simulink model "LPVT_CollectivePitch_50"  (R2018a)
settings: Solver=FixedStepAuto  StartTime=0.0  StopTime=FA.TMax  FixedStep=FA.DT  RelTol=1e-3  EnableMultiTasking=on
undefined symbols (not defined in the file or in its folder): Control, DiscIntNeverNeededParam, FA, OutList, Parameters, PitchControlParams, rpm2radps, S_ConstTq, S_LowBPLim, strmatch, TorqueControlParams
libraries: simulink_extras x1
settings Model: ExtModeTrigMode=oneshot  ExtModeArmWhenConnect=off  Creator=Dana Martin  LastModifiedBy=dmartin
settings DataIOCC: SaveFormat=Array  SaveOutput=off  InspectSignalLogs=on  SignalLoggingName=sigsOut  OutputTimes=[0:500]/50
settings OptimizationCC: BooleanDataType=off  ExpressionDepthLimit=2147483647  InitFltsAndDblsToZero=on  LifeSpan=inf
settings DebuggingCC: SignalRangeChecking=warning  AlgebraicLoopMsg=error  SaveWithParameterizedLinksMsg=none  UnderspecifiedInitializationDetection=Classic  MergeDetectMultiDrivingBlocksExec=none  SignalResolutionControl=TryResolveAllWithWarning  TimeAdjustmentMsg=warning  MultiTaskDSMMsg=warning  MultiTaskCondExecSysMsg=warning  ParameterUnderflowMsg=warning  UnderSpecifiedDataTypeMsg=warning  UnnecessaryDatatypeConvMsg=warning  VectorMatrixConversionMsg=warning  FcnCallInpInsideContextMsg=warning  SignalLabelMismatchMsg=warning  SFcnCompatibilityMsg=warning  UniqueDataStoreMsg=warning  AllowSymbolicDim=off  ModelReferenceIOMsg=warning  ModelReferenceVersionMismatchMessage=warning  ModelReferenceIOMismatchMessage=warning  StateNameClashWarn=warning  StrictBusMsg=WarnOnBusTreatedAsVector  NonBusSignalsTreatedAsBus=warning  SFUnexpectedBacktrackingDiag=warning  SFNoUnconditionalDefaultTransitionDiag=warning  SFExecutionAtInitializationDiag=none
settings HardwareCC: ProdBitPerPointer=32  ProdBitPerSizeT=32  ProdBitPerPtrDiffT=32  ProdLargestAtomicFloat=None  ProdIntDivRoundTo=Undefined  ProdEndianess=Unspecified  ProdWordSize=32  ProdHWDeviceType=32-bit Generic  TargetBitPerPointer=64  TargetBitPerSizeT=64  TargetBitPerPtrDiffT=64  TargetLongLongMode=on  TargetIntDivRoundTo=Zero  TargetEndianess=LittleEndian  TargetWordSize=64  TargetHWDeviceType=MATLAB Host  ProdEqTarget=off
settings ModelReferenceCC: PropagateSignalLabelsOutOfModel=off
settings CodeAppCC: StateflowObjectComments=on
settings GRTTargetCC: TargetFcnLib=ansi_tfl_tmw.mat  TargetLangStandard=C89/C90 (ANSI)  ModelReferenceCompliant=off  GeneratePreprocessorConditionals=Disable all  CombineOutputUpdateFcns=off  GRTInterface=on
settings ConfigComp: CovMetricSettings=dw  CovHtmlReporting=on  CovSaveCumulativeToWorkspaceVar=on  CovSaveSingleToWorkspaceVar=on  CovExternalEMLEnable=off  CovSFcnEnable=off

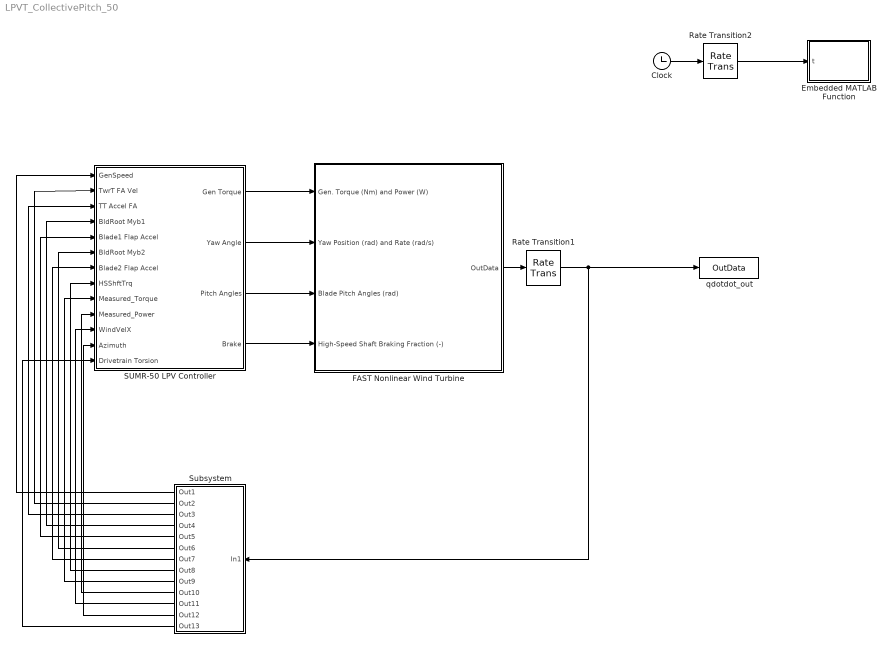
== system LPVT_CollectivePitch_50 ==
  Clock : Clock
  Embedded MATLAB Function : MATLAB Function  TreatAsAtomicUnit=on
  FAST Nonlinear Wind Turbine : Subsystem  mask(FAST Nonlinear Wind Turbine){}
      mask help: This block contains the FAST S-Function.
      mask init:
      | clear FAST_SFunc
  Rate Transition1 : RateTransition
  Rate Transition2 : RateTransition
  SUMR-50 LPV Controller : Subsystem
  Subsystem : Subsystem
  qdotdot_out : ToWorkspace  VariableName=OutData  SaveFormat=Structure With Time  SampleTime=-1
  wires:
  SUMR-50 LPV Controller/1(Gen Torque) -> FAST Nonlinear Wind Turbine/1(Gen. Torque (Nm) and Power (W))
  SUMR-50 LPV Controller/3(Pitch Angles) -> FAST Nonlinear Wind Turbine/3(Blade Pitch Angles (rad))
  SUMR-50 LPV Controller/2(Yaw Angle) -> FAST Nonlinear Wind Turbine/2(Yaw Position (rad) and Rate (rad/s))
  SUMR-50 LPV Controller/4(Brake) -> FAST Nonlinear Wind Turbine/4(High-Speed Shaft Braking Fraction (-))
  Rate Transition1/1 -> Subsystem/1(In1), qdotdot_out/1
  FAST Nonlinear Wind Turbine/1(OutData) -> Rate Transition1/1
  Subsystem/1(Out1) -> SUMR-50 LPV Controller/1(GenSpeed)
  Subsystem/2(Out2) -> SUMR-50 LPV Controller/2(TwrT FA Vel)
  Subsystem/3(Out3) -> SUMR-50 LPV Controller/3(TT Accel FA)
  Subsystem/4(Out4) -> SUMR-50 LPV Controller/4(BldRoot Myb1)
  Subsystem/5(Out5) -> SUMR-50 LPV Controller/5(Blade1 Flap Accel)
  Subsystem/6(Out6) -> SUMR-50 LPV Controller/6(BldRoot Myb2)
  Subsystem/7(Out7) -> SUMR-50 LPV Controller/7(Blade2 Flap Accel)
  Subsystem/8(Out8) -> SUMR-50 LPV Controller/8(HSShftTrq)
  Subsystem/9(Out9) -> SUMR-50 LPV Controller/9(Measured_Torque)
  Subsystem/10(Out10) -> SUMR-50 LPV Controller/10(Measured_Power)
  Subsystem/11(Out11) -> SUMR-50 LPV Controller/11(WindVelX)
  Subsystem/12(Out12) -> SUMR-50 LPV Controller/12(Azimuth)
  Clock/1 -> Rate Transition2/1
  Rate Transition2/1 -> Embedded MATLAB Function/1(t)
  Subsystem/13(Out13) -> SUMR-50 LPV Controller/13(Drivetrain Torsion)

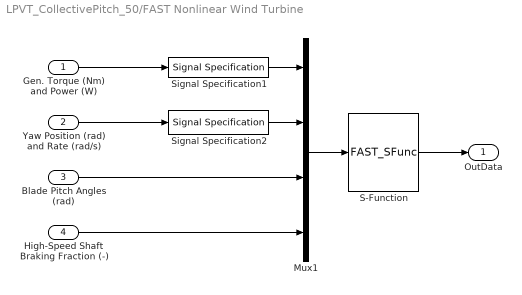
== system LPVT_CollectivePitch_50/FAST Nonlinear Wind Turbine ==
  Gen. Torque (Nm) and Power (W) : Inport
  Yaw Position (rad) and Rate (rad/s) : Inport  Port=2
  Blade Pitch Angles (rad) : Inport  Port=3
  High-Speed Shaft Braking Fraction (-) : Inport  Port=4
  Mux1 : Mux
  S-Function : S-Function  FunctionName=FAST_SFunc  Parameters=FAST_InputFileName, FA.TMax, 0  SFunctionDeploymentMode=off  EnableBusSupport=off
  Signal Specification1 : SignalSpecification  OutDataTypeStr=double  Dimensions=2
  Signal Specification2 : SignalSpecification  OutDataTypeStr=double  Dimensions=2
  OutData : Outport
  wires:
  Gen. Torque (Nm) and Power (W)/1 -> Signal Specification1/1
  S-Function/1 -> OutData/1
  Mux1/1 -> S-Function/1
  Blade Pitch Angles (rad)/1 -> Mux1/3
  Yaw Position (rad) and Rate (rad/s)/1 -> Signal Specification2/1
  Signal Specification1/1 -> Mux1/1
  Signal Specification2/1 -> Mux1/2
  High-Speed Shaft Braking Fraction (-)/1 -> Mux1/4

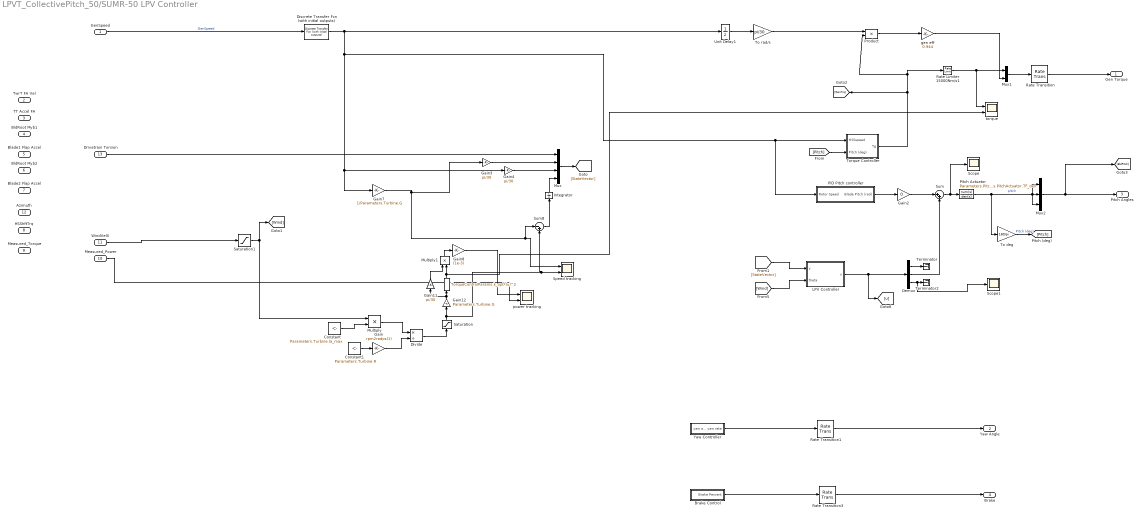
== system LPVT_CollectivePitch_50/SUMR-50 LPV Controller ==
  GenSpeed : Inport
  TwrT FA Vel : Inport  Port=2
  TT Accel FA : Inport  Port=3
  BldRoot Myb1 : Inport  Port=4
  Blade1 Flap Accel : Inport  Port=5
  BldRoot Myb2 : Inport  Port=6
  Blade2 Flap Accel : Inport  Port=7
  HSShftTrq : Inport  Port=8
  Measured_Torque : Inport  Port=9
  Measured_Power : Inport  Port=10
  WindVelX : Inport  Port=11
  Azimuth : Inport  Port=12
  Drivetrain Torsion : Inport  Port=13
  " " : Fcn  Expr=TorqueControlParams.k_opt*(u)^2
  Brake Control : Subsystem
  Constant : Constant  Value=Parameters.Turbine.la_max  SampleTime=FA.DT
  Constant1 : Constant  Value=Parameters.Turbine.R
  Demux : Demux  Outputs=3
  Discrete Transfer Fcn (with initial outputs) : simulink_extras/Additional Discrete/Discrete Transfer Fcn (with initial outputs)  N=Parameters.LPF.LPnum  D=Parameters.LPF.LPden  U0=Parameters.Turbine.IC.Wg  Y0=Parameters.Turbine.IC.Wg  TS=FA.DT
      settings: SourceProductName=Simulink  SourceProductBaseCode=SL
  Divide : Product  Inputs=*/
  Gain : Gain  Gain=rpm2radps(1)
  Gain11 : Gain  Gain=pi/30
  Gain12 : Gain  Gain=Parameters.Turbine.G
  Gain2 : Gain  Gain=0
  Gain3 : Gain  Gain=pi/30
  Gain4 : Gain  Gain=pi/30
  Gain7 : Gain  Gain=1/Parameters.Turbine.G
  Gain8 : Gain  Gain=(1e-3)
  Integrator : Integrator
  LPV Controller : Subsystem  TreatAsAtomicUnit=on
      settings: MinAlgLoopOccurrences=on
  Multiply : Product
  Multiply1 : Product
  Mux : Mux
  Mux1 : Mux  Inputs=2
  Mux2 : Mux  Inputs=3
  PID Pitch controller : Subsystem
      settings: MinAlgLoopOccurrences=on
  Pitch Actuator : TransferFcn  Numerator=Parameters.PitchActuator.TF_num  Denominator=Parameters.PitchActuator.TF_den
  Product : Product  RndMeth=Zero
  Rate Limiter 15000Nm/s1 : RateLimiter  RisingSlewLimit=15000  FallingSlewLimit=-15000  SampleTimeMode=inherited
  Rate Transition : RateTransition  InitialCondition=Parameters.Turbine.IC.Tg
  Rate Transition1 : RateTransition
  Rate Transition3 : RateTransition
  Saturation : Saturate  UpperLimit=Parameters.Turbine.wr_rated  LowerLimit=0
  Saturation1 : Saturate  UpperLimit=25  LowerLimit=0
  Scope : Scope
  Scope1 : Scope
  Speed tracking : Scope  NumInputPorts=2
  Sum : Sum  Inputs=|++
  Sum8 : Sum  Inputs=|-+
  Terminator : Terminator
  Terminator2 : Terminator
  To deg : Gain  Gain=180/pi
  To rad/s : Gain  Gain=pi/30
  Torque Controller : Subsystem
  Unit Delay1 : UnitDelay  InitialCondition=Parameters.Turbine.IC.Wg  SampleTime=FA.DT
  Yaw Controller : Subsystem
  gen eff : Gain  Gain=0.944
  power tracking : Scope  NumInputPorts=2
  torque : Scope  NumInputPorts=2
  Gen Torque : Outport
  Yaw Angle : Outport  Port=2
  Pitch Angles : Outport  Port=3
  Brake : Outport  Port=4
  wires:
  Mux1/1 -> Rate Transition/1
  Product/1 -> gen eff/1
  Unit Delay1/1 -> To rad/s/1
  To rad/s/1 -> Product/1
  gen eff/1 -> Mux1/2
  GenSpeed/1 -> Discrete Transfer Fcn (with initial outputs)/1  "GenSpeed"
  Yaw Controller/1(yaw and yaw rate) -> Rate Transition1/1
  Brake Control/1(Brake Percent) -> Rate Transition3/1
  Rate Transition3/1 -> Brake/1
  Rate Transition1/1 -> Yaw Angle/1
  Constant/1 -> Multiply/2
  Multiply/1 -> Divide/1
  Constant1/1 -> Gain/1
  Gain/1 -> Divide/2
  LPV Controller/1(u) -> Demux/1, [u]
  Mux2/1 -> [BldPitch], Pitch Angles/1
  Rate Transition/1 -> Gen Torque/1
  WindVelX/1 -> Saturation1/1
  Multiply1/1 -> Gain8/1
  Gain11/1 -> Multiply1/1
  Divide/1 -> Saturation/1
  Gain12/1 -> Gain11/1, " "/1
  Saturation1/1 -> [Wind], Multiply/1
  Measured_Power/1 -> power tracking/2
  " "/1 -> torque/2, Multiply1/2
  Pitch Actuator/1 -> To deg/1, Mux2/1, Mux2/2, Mux2/3  "pitch"
  Rate Limiter 15000Nm/s1/1 -> Mux1/1, torque/1
  [StateVector] -> LPV Controller/1(y)
  [Wind] -> LPV Controller/2(theta)
  Gain8/1 -> power tracking/1
  Mux/1 -> [StateVector]
  To deg/1 -> [Pitch]  "Pitch (deg)"
  [Pitch] -> Torque Controller/2(Pitch (deg))
  Demux/1 -> Terminator/1
  Sum/1 -> Scope/1, Pitch Actuator/1
  PID Pitch controller/1(Blade Pitch (rad)) -> Gain2/1
  Gain2/1 -> Sum/1
  Saturation/1 -> Gain12/1, Sum8/2, Speed tracking/2
  Discrete Transfer Fcn (with initial outputs)/1 -> PID Pitch controller/1(Rotor Speed), Torque Controller/1(HSSspeed), Gain7/1, Gain4/1, Unit Delay1/1
  Demux/2 -> Sum/2
  Drivetrain Torsion/1 -> Mux/1
  Integrator/1 -> Mux/4
  Sum8/1 -> Integrator/1
  Gain4/1 -> Mux/3
  Gain3/1 -> Mux/2
  Demux/3 -> Scope1/1, Terminator2/1
  Gain7/1 -> Gain3/1, Sum8/1, Speed tracking/1
  Torque Controller/1(Tg) -> [GenTrq], Product/2, Rate Limiter 15000Nm/s1/1

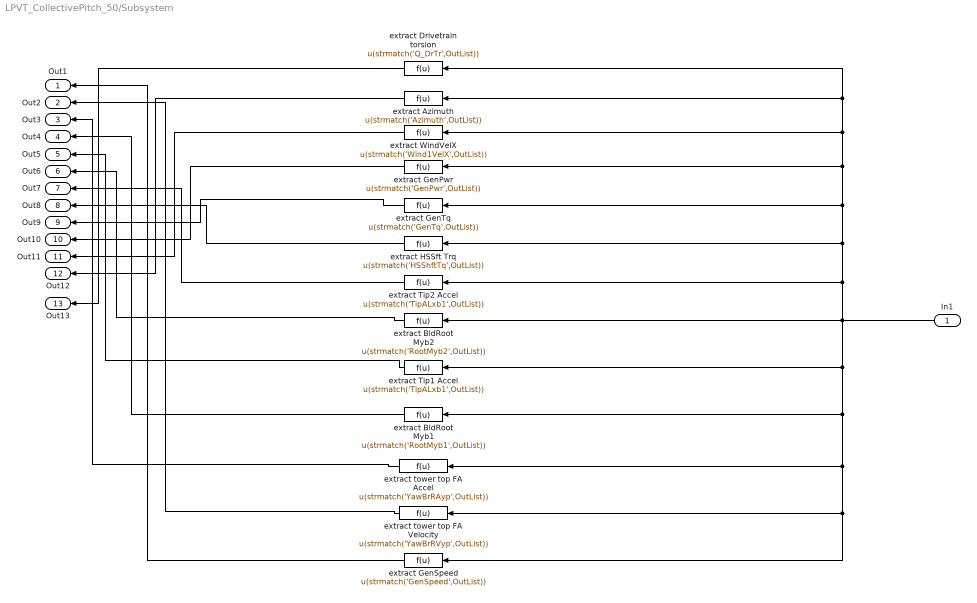
== system LPVT_CollectivePitch_50/Subsystem ==
  In1 : Inport
  extract Azimuth : Fcn  Expr=u(strmatch('Azimuth',OutList))
  extract BldRoot Myb1 : Fcn  Expr=u(strmatch('RootMyb1',OutList))
  extract BldRoot Myb2 : Fcn  Expr=u(strmatch('RootMyb2',OutList))
  extract Drivetrain torsion : Fcn  Expr=u(strmatch('Q_DrTr',OutList))
  extract GenPwr : Fcn  Expr=u(strmatch('GenPwr',OutList))
  extract GenSpeed : Fcn  Expr=u(strmatch('GenSpeed',OutList))
  extract GenTq : Fcn  Expr=u(strmatch('GenTq',OutList))
  extract HSSft Trq : Fcn  Expr=u(strmatch('HSShftTq',OutList))
  extract Tip1 Accel : Fcn  Expr=u(strmatch('TipALxb1',OutList))
  extract Tip2 Accel : Fcn  Expr=u(strmatch('TipALxb1',OutList))
  extract WindVelX : Fcn  Expr=u(strmatch('Wind1VelX',OutList))
  extract tower top FA Accel : Fcn  Expr=u(strmatch('YawBrRAyp',OutList))
  extract tower top FA Velocity : Fcn  Expr=u(strmatch('YawBrRVyp',OutList))
  Out1 : Outport
  Out2 : Outport  Port=2
  Out3 : Outport  Port=3
  Out4 : Outport  Port=4
  Out5 : Outport  Port=5
  Out6 : Outport  Port=6
  Out7 : Outport  Port=7
  Out8 : Outport  Port=8
  Out9 : Outport  Port=9
  Out10 : Outport  Port=10
  Out11 : Outport  Port=11
  Out12 : Outport  Port=12
  Out13 : Outport  Port=13
  wires:
  extract WindVelX/1 -> Out11/1
  extract GenTq/1 -> Out9/1
  In1/1 -> extract Drivetrain torsion/1, extract Azimuth/1, extract WindVelX/1, extract GenPwr/1, extract GenTq/1, extract HSSft Trq/1, extract Tip2 Accel/1, extract BldRoot Myb2/1, extract Tip1 Accel/1, extract BldRoot Myb1/1, extract tower top FA Velocity/1, extract GenSpeed/1, extract tower top FA Accel/1
  extract GenPwr/1 -> Out10/1
  extract Tip1 Accel/1 -> Out5/1
  extract HSSft Trq/1 -> Out8/1
  extract tower top FA Velocity/1 -> Out2/1
  extract tower top FA Accel/1 -> Out3/1
  extract Tip2 Accel/1 -> Out7/1
  extract Azimuth/1 -> Out12/1
  extract BldRoot Myb2/1 -> Out6/1
  extract GenSpeed/1 -> Out1/1
  extract BldRoot Myb1/1 -> Out4/1
  extract Drivetrain torsion/1 -> Out13/1

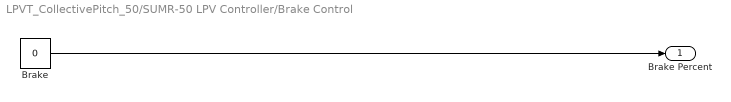
== system LPVT_CollectivePitch_50/SUMR-50 LPV Controller/Brake Control ==
  Brake : Constant  Value=0  SampleTime=-1
  Brake Percent : Outport
  wires:
  Brake/1 -> Brake Percent/1

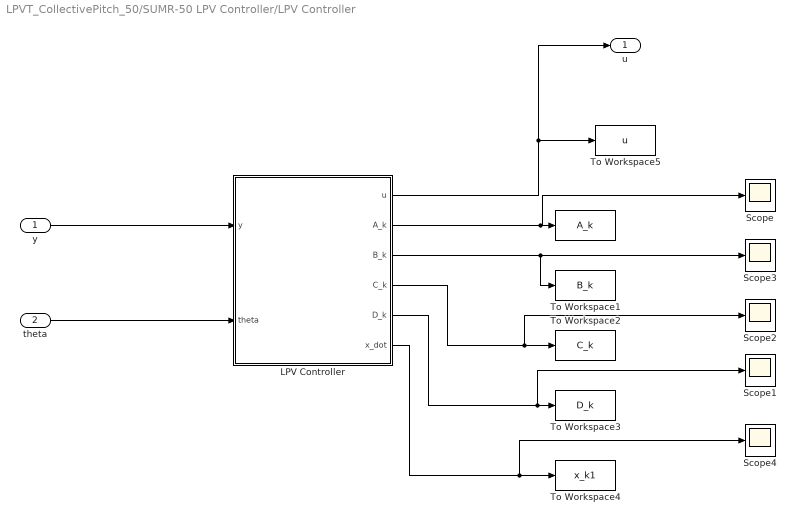
== system LPVT_CollectivePitch_50/SUMR-50 LPV Controller/LPV Controller ==
  y : Inport
  theta : Inport  Port=2
  " " : ToWorkspace  VariableName=A_k  SaveFormat=Structure With Time  SampleTime=-1
      settings: Decimation=3
  LPV Controller : MATLAB Function  TreatAsAtomicUnit=on  SystemSampleTime=FA.DT
      settings: MinAlgLoopOccurrences=on
  Scope{,1..4} (5 alike) : Scope
  To Workspace1 : ToWorkspace  VariableName=B_k  SaveFormat=Structure With Time  SampleTime=-1
      settings: Decimation=3
  To Workspace2 : ToWorkspace  VariableName=C_k  SaveFormat=Structure With Time  SampleTime=-1
      settings: Decimation=3
  To Workspace3 : ToWorkspace  VariableName=D_k  SaveFormat=Structure With Time  SampleTime=-1
      settings: Decimation=3
  To Workspace4 : ToWorkspace  VariableName=x_k1  SaveFormat=Structure With Time  SampleTime=-1
      settings: Decimation=3
  To Workspace5 : ToWorkspace  VariableName=u  SaveFormat=Structure With Time  SampleTime=-1
      settings: Decimation=3
  u : Outport
  wires:
  theta/1 -> LPV Controller/2(theta)
  y/1 -> LPV Controller/1(y)
  LPV Controller/3(B_k) -> Scope3/1, To Workspace1/1
  LPV Controller/2(A_k) -> Scope/1, " "/1
  LPV Controller/5(D_k) -> Scope1/1, To Workspace3/1
  LPV Controller/1(u) -> To Workspace5/1, u/1
  LPV Controller/4(C_k) -> Scope2/1, To Workspace2/1
  LPV Controller/6(x_dot) -> Scope4/1, To Workspace4/1

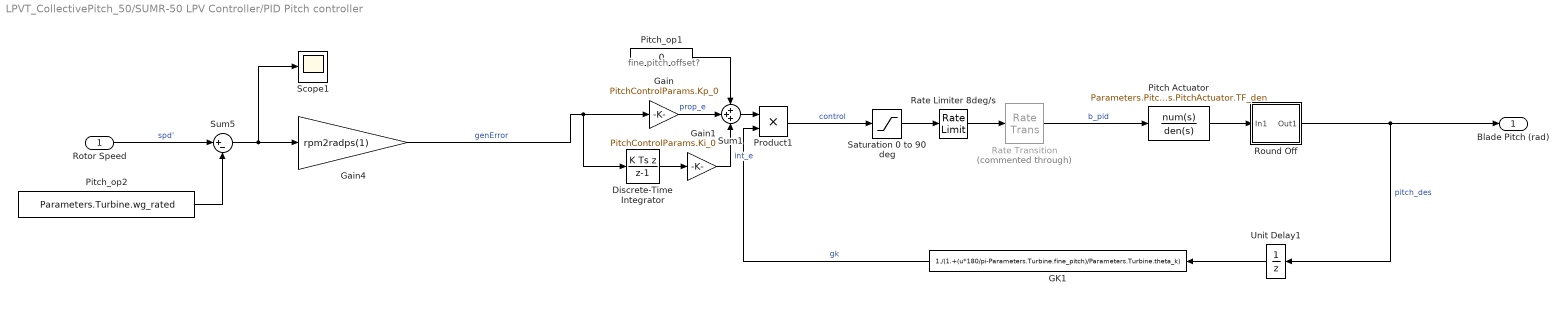
== system LPVT_CollectivePitch_50/SUMR-50 LPV Controller/PID Pitch controller ==
  note: fine pitch offset?
  Rotor Speed : Inport
  Discrete-Time Integrator : DiscreteIntegrator  IntegratorMethod=Integration: Backward Euler  gainval=1  InitialCondition=deg2rad(Parameters.Turbine.fine_pitch)/(PitchControlParams.Ki_0)/(1./(1.+deg2rad(Parameters.Turbine.fine_pitch)/PitchControlParams.theta_k))  SampleTime=Control.DT  LimitOutput=on  UpperSaturationLimit=5*1.570796/(PitchControlParams.Ki_0)/(1./(1.+1.570796/PitchControlParams.theta_k))  LowerSaturationLimit=deg2rad(Parameters.Turbine.fine_pitch)/(PitchControlParams.Ki_0)/(1./(1.+deg2rad(Parameters.Turbine.fine_pitch)/PitchControlParams.theta_k))  ICPrevOutput=DiscIntNeverNeededParam  ICPrevScaledInput=DiscIntNeverNeededParam
  GK1 : Fcn  Expr=1./(1.+(u*180/pi-Parameters.Turbine.fine_pitch)/Parameters.Turbine.theta_k)
  Gain : Gain  Gain=PitchControlParams.Kp_0
  Gain1 : Gain  Gain=PitchControlParams.Ki_0
  Gain4 : Gain  Gain=rpm2radps(1)
  Pitch Actuator : TransferFcn  Numerator=Parameters.PitchActuator.TF_num  Denominator=Parameters.PitchActuator.TF_den
  Pitch_op1 : Constant  Value=0  SampleTime=Control.DT
  Pitch_op2 : Constant  Value=Parameters.Turbine.wg_rated  SampleTime=Control.DT
  Product1 : Product  RndMeth=Zero
  Rate Limiter 8deg/s : RateLimiter  RisingSlewLimit=18*pi/180  FallingSlewLimit=-18*pi/180  SampleTimeMode=inherited  InitialCondition=deg2rad(0)
  Rate Transition : RateTransition  Commented=through
  Round Off : Subsystem
  Saturation 0 to 90 deg : Saturate  UpperLimit=90*pi/180  LowerLimit=deg2rad(Parameters.Turbine.fine_pitch)
  Scope1 : Scope
  Sum1 : Sum  Inputs=+++
  Sum5 : Sum  Inputs=|+-  SaturateOnIntegerOverflow=on  InputSameDT=on  OutDataTypeStr=Inherit: Same as first input
  Unit Delay1 : UnitDelay  InitialCondition=Parameters.Turbine.IC.Wg  SampleTime=Control.DT
  Blade Pitch (rad) : Outport
  wires:
  Pitch_op2/1 -> Sum5/2
  Rotor Speed/1 -> Sum5/1  "spd'"
  Discrete-Time Integrator/1 -> Gain1/1
  Gain/1 -> Sum1/2  "prop_e"
  Pitch_op1/1 -> Sum1/1
  Gain1/1 -> Sum1/3  "int_e"
  Sum1/1 -> Product1/1
  Saturation 0 to 90 deg/1 -> Rate Limiter 8deg/s/1
  Rate Transition/1 -> Pitch Actuator/1  "b_pid"
  Rate Limiter 8deg/s/1 -> Rate Transition/1
  Sum5/1 -> Scope1/1, Gain4/1
  Round Off/1(Out1) -> Blade Pitch (rad)/1, Unit Delay1/1  "pitch_des"
  Product1/1 -> Saturation 0 to 90 deg/1  "control"
  Gain4/1 -> Discrete-Time Integrator/1, Gain/1  "genError"
  Pitch Actuator/1 -> Round Off/1(In1)
  GK1/1 -> Product1/2  "gk"
  Unit Delay1/1 -> GK1/1

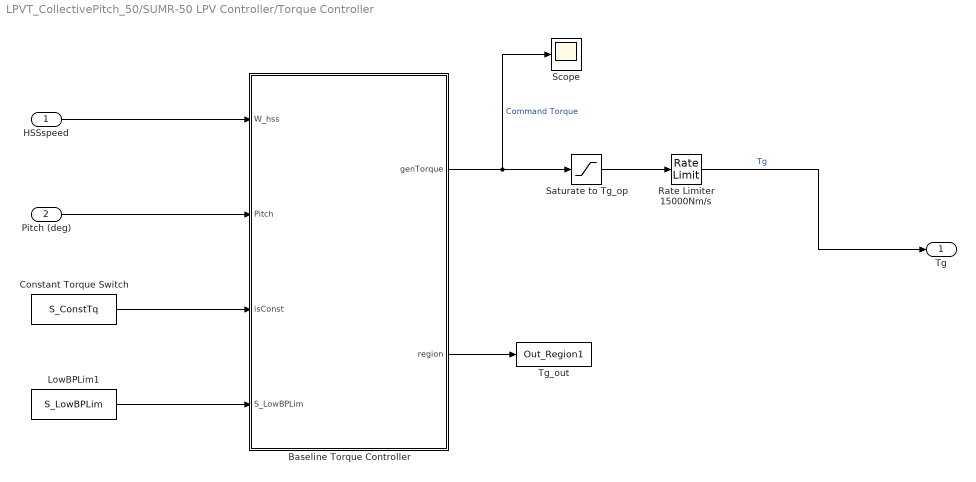
== system LPVT_CollectivePitch_50/SUMR-50 LPV Controller/Torque Controller ==
  HSSspeed : Inport
  Pitch (deg) : Inport  Port=2
  Baseline Torque Controller : MATLAB Function  TreatAsAtomicUnit=on
  Constant Torque Switch : Constant  Value=S_ConstTq  SampleTime=Control.DT
  LowBPLim1 : Constant  Value=S_LowBPLim  SampleTime=Control.DT
  Rate Limiter 15000Nm/s : RateLimiter  RisingSlewLimit=15000  FallingSlewLimit=-15000  SampleTimeMode=inherited
  Saturate to Tg_op : Saturate  UpperLimit=TorqueControlParams.T_rated  LowerLimit=0
  Scope : Scope
  Tg_out : ToWorkspace  VariableName=Out_Region1  SampleTime=-1
      settings: MaxDataPoints=Inf
  Tg : Outport
  wires:
  Saturate to Tg_op/1 -> Rate Limiter 15000Nm/s/1
  Rate Limiter 15000Nm/s/1 -> Tg/1  "Tg"
  Baseline Torque Controller/1(genTorque) -> Saturate to Tg_op/1, Scope/1  "Command Torque"
  Baseline Torque Controller/2(region) -> Tg_out/1
  HSSspeed/1 -> Baseline Torque Controller/1(W_hss)
  Constant Torque Switch/1 -> Baseline Torque Controller/3(isConst)
  LowBPLim1/1 -> Baseline Torque Controller/4(S_LowBPLim)
  Pitch (deg)/1 -> Baseline Torque Controller/2(Pitch)

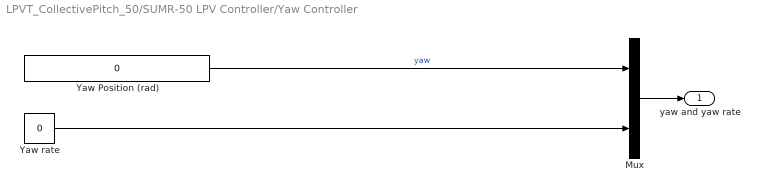
== system LPVT_CollectivePitch_50/SUMR-50 LPV Controller/Yaw Controller ==
  Mux : Mux  Inputs=2
  Yaw Position (rad) : Constant  Value=0  SampleTime=-1
  Yaw rate : Constant  Value=0  SampleTime=-1
  yaw and yaw rate : Outport
  wires:
  Mux/1 -> yaw and yaw rate/1
  Yaw Position (rad)/1 -> Mux/1  "yaw"
  Yaw rate/1 -> Mux/2

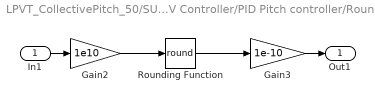
== system LPVT_CollectivePitch_50/SUMR-50 LPV Controller/PID Pitch controller/Round Off ==
  In1 : Inport
  Gain2 : Gain  Gain=1e10
  Gain3 : Gain  Gain=1e-10
  Rounding Function : Rounding  Operator=round
  Out1 : Outport
  wires:
  Gain2/1 -> Rounding Function/1
  Rounding Function/1 -> Gain3/1
  Gain3/1 -> Out1/1
  In1/1 -> Gain2/1

== matlab function LPVT_CollectivePitch_50/SUMR-50 LPV Controller/LPV Controller/LPV Controller ==
  data: y input; theta input; u output; A_k output; B_k output; C_k output; D_k output; x_dot output
function [u,  A_k, B_k, C_k, D_k, x_dot]   = LPVController(y, theta)
% coder.extrinsic('trapz')

persistent x_kp;

if isempty(x_kp)
    x_kp = zeros(2,1); 
end
K_bar = [      0.000000000000000000000000048366597452873417656909046829519*theta^3 - 0.0000000000000000000000034141603475377986983932003739181*theta^2 + 0.000000000000000000000079893451476199432434659916811555*theta + 144363883517824.0,    0.0000000000000000000096789979496213551201491173022877*theta^3 - 0.00000000000000000075138126074754960441287880185147*theta^2 + 0.000000000000000019549680656633766500236579187554*theta - 401602695420160.0,        - 0.000000000000000000000000068800936898101181323695460984235*theta^3 + 0.00000000000000000000000486445933252241550691091003065*theta^2 - 0.00000000000000000000011405804811803262359045484530227*theta + 103345618276400.0,       - 0.0000000000000000000027384638939477589187146455519834*theta^3 + 0.00000000000000000015825183681684529475041265871359*theta^2 - 0.0000000000000000026914565514280752772989572904826*theta + 89335437525536.0,                      -142390141410656.0,        -998798994893.125;
                                      - 0.000000000000021306154871489412796778468704739*theta^3 + 0.0000000000015039848356422248284355779805559*theta^2 - 0.00000000003519416994400103582604495515429*theta - 380735404819742720.0,                                     - 0.0000000042637324140155680347874511681994*theta^3 + 0.00000033099383359809150806363220453932*theta^2 - 0.0000086119046138026511538754448338295*theta - 384237041946560.0,                                        0.000000000000030307763912535316262650516549982*theta^3 - 0.0000000000021428615896695765330757848729504*theta^2 + 0.000000000050244147108144839223675508221856*theta - 170446034460114944.0,                                        0.0000000012063312059792228214845366540686*theta^3 - 0.000000069712122032202579642590212216646*theta^2 + 0.0000011856238216979755190072509662969*theta - 150150287328509952.0,                    380735010664218624.0,       -153287910156.8125;
 0.00000000000000000000000000086824813988457424840453546538632*theta^3 - 0.000000000000000000000000061288958230014895865568109911177*theta^2 + 0.0000000000000000000000014341993087429475916657868811635*theta + 492938350426560.0, 0.00000000000000000000017375156426691693268545022218738*theta^3 - 0.000000000000000000013488345600986063672676257308921*theta^2 + 0.00000000000000000035094413829703289641301155347878*theta + 547903552588.375, - 0.0000000000000000000000000012350731420022324587327624393006*theta^3 + 0.000000000000000000000000087323855500099886727719110512806*theta^2 - 0.0000000000000000000000020475016505726569915259550265613*theta + 220711397770816.0, - 0.000000000000000000000049159260879941153989248484603568*theta^3 + 0.0000000000000000000028408420311850819823506178091784*theta^2 - 0.00000000000000000004831541326913238328173397601363*theta + 194435424021216.0,                      -492937991714304.0, 195778215.10076904296875;
           - 0.000000000000000000000004081054099639780652538529460165*theta^3 + 0.00000000000000000000028807842223601879055057353744289*theta^2 - 0.0000000000000000000067412122177708148011572776173208*theta + 584557992064640.0,        - 0.00000000000000000081668995428510217288986510144496*theta^3 + 0.000000000000000063399695989663338879977023446234*theta^2 - 0.0000000000000016495537952228313737079269922858*theta + 372854244360768.0,             0.0000000000000000000000058052532196550408958749226383689*theta^3 - 0.00000000000000000000041045107051133273769583464338754*theta^2 + 0.0000000000000000000096239365467583696539812221688099*theta + 198690604824320.0,              0.00000000000000000023106482344559432515400585352623*theta^3 - 0.000000000000000013352899344349677880003647990623*theta^2 + 0.00000000000000022709845992185658604288250372807*theta + 173251849994944.0,                      -586356159891200.0,         -4668503117911.0;
                                                                                                                                                                                                               13045512707665920.0,                                                                                                                                                                                                14373836424148.0,                                                                                                                                                                                                                 5840994271941632.0,                                                                                                                                                                                                   5145601411204096.0,                    -13045505203230720.0,    5315725970.2431640625;
                                                                                                                                                                                                        18370483.59114837646484375,                                                                                                                                                                                                 5713970330199.0,                                                                                                                                                                                                        -26442606.72623443603515625,                                                                                                                                                                                             -9728272.924530029296875, -0.000002075025962868827511531577556525,         -5665747606912.0];
S1 = 6e-18;                                                                                                
S2 = 6e-18;
A_k             = S1*K_bar(1:2,1:2);
Controller.A_k  = A_k;

B_k             = S2*K_bar(1:2,3:6);
Controller.B_k  = B_k;

C_k             = S1*K_bar(3:5,1:2);
Controller.C_k  = C_k;

D_k             = S2*K_bar(3:5,3:6);
Controller.B_k  = D_k;

x_dot           = A_k*x_kp+B_k*y;
Controller.x_k1 = x_dot;

u               = C_k*x_kp+D_k*y; 

x_kp            = x_dot;

end

== matlab function LPVT_CollectivePitch_50/Embedded MATLAB Function ==
  data: t input
function TellTime(t)

if t==0
    Tsim=t
elseif rem(t,50)==0
    Tsim=t
end

== matlab function LPVT_CollectivePitch_50/SUMR-50 LPV Controller/Torque Controller/Baseline Torque Controller ==
  settings: updateMethod=DISCRETE  sampleTime=Control.DT
  data: W_hss input; Pitch input; genTorque output; isConst input; region output; S_LowBPLim input; TorqueControlParams parameter
function [genTorque, region] = regionSelectTq_Flex( W_hss, Pitch, isConst, S_LowBPLim, TorqueControlParams)
% This block supports an embeddable subset of the MATLAB language.
% See the help menu for details.


%% Assign Constants

wg_rated    = TorqueControlParams.wg_rated;
T_rated     = TorqueControlParams.T_rated;
w2_high     = TorqueControlParams.w2_high;
w1_high     = TorqueControlParams.w1_high;
wg_min      = TorqueControlParams.wg_min;
m2_5        = TorqueControlParams.m2_5;
c2_5        = TorqueControlParams.c2_5;
m1_5        = TorqueControlParams.m1_5;
c1_5        = TorqueControlParams.c1_5;
k_opt       = TorqueControlParams.k_opt;
P0          = TorqueControlParams.P0;
T2_high     = m2_5 * w2_high + c2_5;

%% Switch based on Gen. Speed

if (((S_LowBPLim==0)&&(W_hss >= wg_rated)) || ((S_LowBPLim==1)&&((Pitch >= TorqueControlParams.fine_pitch+1) || (W_hss >= wg_rated)))) %Region 3 calcs
    region=3;
    if (isConst)
        genTorque = T_rated;
    else
        genTorque = 30/pi * P0 / W_hss;
    end
elseif (W_hss >= w2_high)                %Region 2.5
    region=2.5;    
    genTorque = m2_5 * W_hss + c2_5;
    
elseif (W_hss >= w1_high)                    %Region 2
    region=2;
    genTorque = k_opt * W_hss^2;
elseif (W_hss > wg_min)                    %Region 1.5
    region=1.5;
    genTorque = m1_5 * W_hss + c1_5;
else                                    %Region 1
    region=1;
    genTorque = 0;
end
